simulink model "DiodeRectifier_BuckConverter_SecondEdition"  (R2021b)
settings: Solver=VariableStepAuto  StartTime=0.0  StopTime=0.2  MaxStep=1e-5  RelTol=1e-3
libraries: spsMeanLib x9, spsDiodeLib x7, spsSeriesRLCBranchLib x5, spsVoltageMeasurementLib x3, spsCurrentMeasurementLib x3, spsACVoltageSourceLib x3, spsDCVoltageSourceLib x1, spsMosfetLib x1, spsPWMGeneratorDCDCLib x1, spsTHDLib x1, spspowerguiLib x1
settings Model: Creator=Emre Çakmakyurdu  LastModifiedBy=Emre Çakmakyurdu

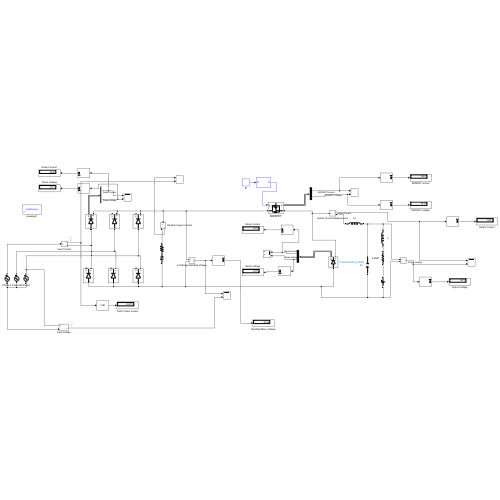
[thumbnail: Simulink's stored preview of the top-level diagram]
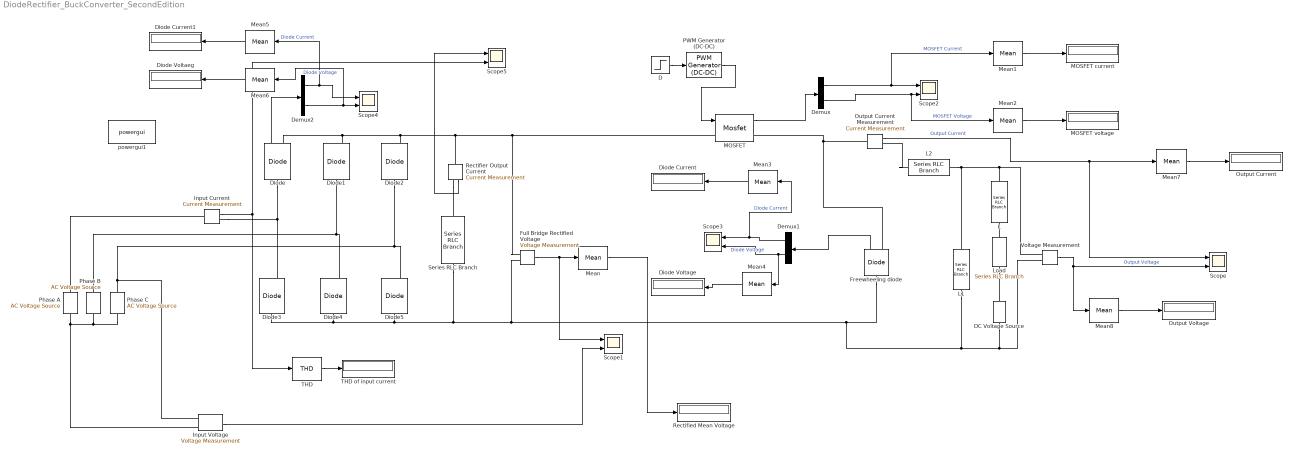
== system DiodeRectifier_BuckConverter_SecondEdition ==
  D : Step  Time=0  Before=0.7695  After=0.7695  SampleTime=0
  DC Voltage Source : spsDCVoltageSourceLib/DC Voltage Source  Amplitude=0.1  Measurements=None
  Demux : Demux  Outputs=2
  Demux1 : Demux  Outputs=2
  Demux2 : Demux  Outputs=2
  Diode{,1..5} (6 alike) : spsDiodeLib/Diode  Ron=0  Lon=0  Vf=0  IC=0  UseSnubber=0  Rs=inf  Cs=0  Measurements=on
  Diode Current : Display
  Diode Current1 : Display
  Diode Voltaeg : Display
  Diode Voltage : Display
  "Freewheeling diode " : spsDiodeLib/Diode  Ron=0  Lon=0  Vf=0  IC=0  UseSnubber=off  Rs=inf  Cs=0  Measurements=on
  Full Bridge Rectified Voltage : spsVoltageMeasurementLib/Voltage Measurement  PhasorSimulation=off  OutputType=Complex  PSBequivalent=0
  Input Current : spsCurrentMeasurementLib/Current Measurement  PhasorSimulation=off  OutputType=Complex  PSBequivalent=0
  Input Voltage : spsVoltageMeasurementLib/Voltage Measurement  PhasorSimulation=off  OutputType=Complex  PSBequivalent=0
  L : spsSeriesRLCBranchLib/Series RLC Branch  LConnTagsString=__new0  RConnTagsString=__new0  BranchType=L  Resistance=0.02  Inductance=24e-3  SetiL0=off  InitialCurrent=0  Capacitance=1e-6  Setx0=off  InitialVoltage=0  Measurements=None
  L1 : spsSeriesRLCBranchLib/Series RLC Branch  LConnTagsString=__new0  RConnTagsString=__new0  BranchType=C  Resistance=0.02  Inductance=24e-3  SetiL0=off  InitialCurrent=0  Capacitance=4.09e-6  Setx0=off  InitialVoltage=0  Measurements=None
  L2 : spsSeriesRLCBranchLib/Series RLC Branch  LConnTagsString=__new0  RConnTagsString=__new0  BranchType=L  Resistance=0.02  Inductance=0.00596  SetiL0=off  InitialCurrent=0  Capacitance=1e-6  Setx0=off  InitialVoltage=0  Measurements=None
  Load : spsSeriesRLCBranchLib/Series RLC Branch  LConnTagsString=__new0  RConnTagsString=__new0  BranchType=R  Resistance=1.07  Inductance=200e-6  SetiL0=off  InitialCurrent=0  Capacitance=400e-6  Setx0=off  InitialVoltage=0  Measurements=None
  MOSFET : spsMosfetLib/Mosfet  Ron=0.1  Lon=0  Rd=0.01  Vfd=0  IC=0  Rs=1e5  Cs=inf  Measurements=on
  MOSFET current : Display
  MOSFET voltage : Display
  Mean{,1..8} (9 alike) : spsMeanLib/Mean  Freq=50  Vinit=0  Ts=0
  Output Current : Display
  Output Current Measurement : spsCurrentMeasurementLib/Current Measurement  PhasorSimulation=off  OutputType=Complex  PSBequivalent=0
  Output Voltage : Display
  PWM Generator (DC-DC) : spsPWMGeneratorDCDCLib/PWM Generator (DC-DC)  Fsw=1e3  Ts=0
  Phase A : spsACVoltageSourceLib/AC Voltage Source  Amplitude=100*sqrt(2)  Phase=0  Frequency=50  SampleTime=0  Measurements=None  BusType=swing  Pref=10e3  Qref=0  Qmin=-inf  Qmax=+inf
  Phase B : spsACVoltageSourceLib/AC Voltage Source  Amplitude=100*sqrt(2)  Phase=-120  Frequency=50  SampleTime=0  Measurements=None  BusType=swing  Pref=10e3  Qref=0  Qmin=-inf  Qmax=+inf
  Phase C : spsACVoltageSourceLib/AC Voltage Source  Amplitude=100*sqrt(2)  Phase=120  Frequency=50  SampleTime=0  Measurements=None  BusType=swing  Pref=10e3  Qref=0  Qmin=-inf  Qmax=+inf
  Rectified Mean Voltage : Display
  Rectifier Output Current : spsCurrentMeasurementLib/Current Measurement  PhasorSimulation=off  OutputType=Complex  PSBequivalent=0
  Scope{,1..5} (6 alike) : Scope  NumInputPorts=2
  Series RLC Branch : spsSeriesRLCBranchLib/Series RLC Branch  LConnTagsString=__new0  RConnTagsString=__new0  BranchType=RC  Resistance=0.0001  Inductance=1e-3  SetiL0=off  InitialCurrent=0  Capacitance=47e-6  Setx0=off  InitialVoltage=0  Measurements=None
  THD : spsTHDLib/THD  Freq=60  Ts=0
      settings: SourceProductBaseCode=PS
  THD of input current : Display
  Voltage Measurement : spsVoltageMeasurementLib/Voltage Measurement  PhasorSimulation=off  OutputType=Complex  PSBequivalent=0
  powergui1 : spspowerguiLib/powergui  Priority=1  SimulationMode=Continuous  SampleTime=50e-6  frequency=60  Iterations=50  frequencyindice=50  Pbase=100e6  ErrMax=1e-4  UnitsV=kV  UnitsW=MW  buscounter=0  FunctionMessages=off  echomessages=off  EnableUseOfTLC=off  CurrentSourceSwitches=off  DisableSnubberDevices=off  DisableRonSwitches=off  DisableVfSwitches=off  DisplayEquations=off  AutomaticDiscreteSolvers=off  SolverType=Tustin/Backward Euler (TBE)  Interpol=off  ExternalGateDelay=off  methode=off  Ts=100  x0status=blocks  SPID=on  SwTol=0  HookPort=off  NonlinearTolerance=1e-4  nMaxIteration=100  ContinueOnMaxIteration=off  RestoreLinks=warning  ResistiveCurrentMeasurement=off  Frange=[0:2:500]  Ylog=off  Xlog=on  ShowGrid=off  save=off  variable=ZData  structure=0  ZoomFFT=off  StartTime=0.0  cycles=1  DisplayStyle=1  fundamental=60  FreqAxis=off  MaxFrequency=1000  frequencyindicesteady=1  RmsSteady=1  display=off
  wires:
  MOSFET/1 -> Demux/1
  Demux/2 -> Mean2/1, Scope2/2  "MOSFET Voltage"
  PWM Generator (DC-DC)/1 -> MOSFET/1
  Demux1/1 -> Mean3/1, Scope3/1  "Diode Current"
  Demux/1 -> Mean1/1, Scope2/1  "MOSFET Current"
  "Freewheeling diode "/1 -> Demux1/1
  D/1 -> PWM Generator (DC-DC)/1
  Demux1/2 -> Mean4/1, Scope3/2  "Diode Voltage"
  Rectifier Output Current/1 -> Scope5/1
  Diode/1 -> Demux2/1
  Demux2/1 -> Mean5/1, Scope4/1  "Diode Current"
  Input Voltage/1 -> Scope1/2
  THD/1 -> THD of input current/1
  Full Bridge Rectified Voltage/1 -> Scope1/1, Mean/1
  Demux2/2 -> Mean6/1, Scope4/2  "Diode Voltage"
  Input Current/1 -> Scope5/2, THD/1
  Mean/1 -> Rectified Mean Voltage/1
  Mean1/1 -> MOSFET current/1
  Mean2/1 -> MOSFET voltage/1
  Mean3/1 -> Diode Current/1
  Mean4/1 -> Diode Voltage/1
  Mean5/1 -> Diode Current1/1
  Mean6/1 -> Diode Voltaeg/1
  Mean7/1 -> Output Current/1
  Output Current Measurement/1 -> Scope/1, Mean7/1  "Output Current"
  Mean8/1 -> Output Voltage/1
  Voltage Measurement/1 -> Mean8/1, Scope/2  "Output Voltage"
  connections:
  Load/RConn1 -- DC Voltage Source/RConn1
  Output Current Measurement/LConn1 -- MOSFET/RConn1 -- "Freewheeling diode "/RConn1
  Diode2/LConn1 -- Diode5/RConn1 -- Input Voltage/LConn1 -- Phase C/RConn1
  DC Voltage Source/LConn1 -- L1/RConn1 -- Series RLC Branch/RConn1 -- Diode5/LConn1 -- Diode3/LConn1 -- Diode4/LConn1 -- Full Bridge Rectified Voltage/LConn2 -- "Freewheeling diode "/LConn1 -- Voltage Measurement/LConn2
  Phase B/LConn1 -- Phase A/LConn1 -- Input Voltage/LConn2 -- Phase C/LConn1
  Diode4/RConn1 -- Phase B/RConn1 -- Diode1/LConn1
  Diode2/RConn1 -- Full Bridge Rectified Voltage/LConn1 -- MOSFET/LConn1 -- Rectifier Output Current/LConn1 -- Diode/RConn1 -- Diode1/RConn1
  Diode3/RConn1 -- Diode/LConn1 -- Input Current/RConn1
  Rectifier Output Current/RConn1 -- Series RLC Branch/LConn1
  Phase A/RConn1 -- Input Current/LConn1
  L2/RConn1 -- Output Current Measurement/RConn1
  L1/LConn1 -- L2/LConn1 -- L/RConn1 -- Voltage Measurement/LConn1
  Load/LConn1 -- L/LConn1
